simulink model "ServoTest"  (R2018a)
settings: Solver=VariableStepAuto  StartTime=0.0  StopTime=300  RelTol=1e-3
values from neighbouring files (symbols this model uses):
  s = mean(abs(present_speed.data))    [RunServoTest.m]
libraries: sm_lib x4, nesl_utility x4, powerlib_meascontrol x1
settings Model: Creator=matt  LastModifiedBy=matt
settings SolverCC: AlgebraicLoopSolver=LineSearch

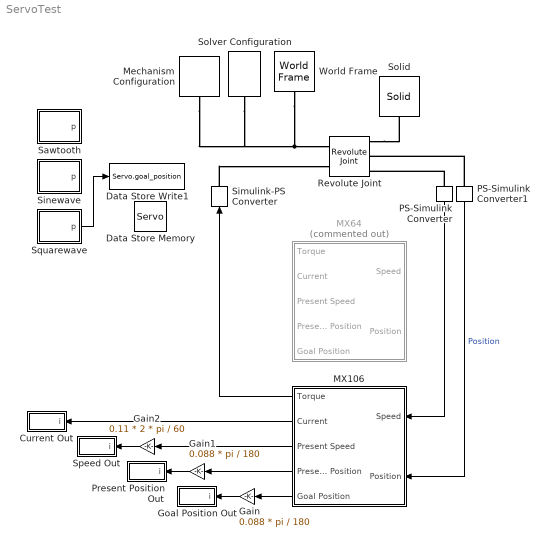
== system ServoTest ==
  Current Out : Subsystem
  Data Store Memory : DataStoreMemory  DataStoreName=Servo  ReadBeforeWriteMsg=warning  WriteAfterWriteMsg=warning  WriteAfterReadMsg=warning  InitialValue=MX64_default  ShowAdditionalParam=off  OutDataTypeStr=Bus: MX64_bus
  Data Store Write1 : DataStoreWrite  DataStoreName=Servo  DataStoreElements=Servo.goal_position
  Gain : Gain  Gain=0.088 * pi / 180
  Gain1 : Gain  Gain=0.088 * pi / 180
  Gain2 : Gain  Gain=0.11 * 2 * pi / 60
  Goal Position Out : Subsystem
  MX106 : Subsystem
  MX64 : Subsystem  Commented=on
  Mechanism Configuration : sm_lib/Utilities/Mechanism Configuration  UniformGravity=Constant  GravityVector=[0 0 0]  GravityUnits=m/s^2  LinearizationDelta=0.001
  PS-Simulink Converter : nesl_utility/PS-Simulink Converter  PhysicalDomain=network_engine_domain  SubClassName=ps_output  LeftPortType=input  RightPortType=output  PseudoPeriodic=off  Frequencies=[]  Unit=rad/s  AffineConversion=off
  PS-Simulink Converter1 : nesl_utility/PS-Simulink Converter  PhysicalDomain=network_engine_domain  SubClassName=ps_output  LeftPortType=input  RightPortType=output  PseudoPeriodic=off  Frequencies=[]  Unit=rad  AffineConversion=off
  Present Position Out : Subsystem
  Revolute Joint : sm_lib/Joints/Revolute Joint  SenseConstraintForce=off  SenseConstraintForceX=off  SenseConstraintForceY=off  SenseConstraintForceZ=off  SenseConstraintTorque=off  SenseConstraintTorqueX=off  SenseConstraintTorqueY=off  SenseConstraintTorqueZ=off  SenseTotalForce=off  SenseTotalForceX=off  SenseTotalForceY=off  SenseTotalForceZ=off  SenseTotalTorque=off  SenseTotalTorqueX=off  SenseTotalTorqueY=off  SenseTotalTorqueZ=off  CompositeWrenchDir=FollowerOnBase  CompositeWrenchFrame=BaseFrame  EquilibriumPosition=0  EquilibriumPositionUnits=deg  SpringStiffness=0  SpringStiffnessUnits=N*m/deg  DampingCoefficient=0  DampingCoefficientUnits=N*m/(rad/s)  TorqueActuationMode=InputTorque  MotionActuationMode=ComputedMotion  SensePosition=on  SenseVelocity=on  SenseAcceleration=off  SenseTorqueForce=off  PositionTargetSpecify=on  PositionTargetPriority=High  PositionTargetValue=MX64_init_position  PositionTargetValueUnits=deg  VelocityTargetSpecify=on  VelocityTargetPriority=High  VelocityTargetValue=MX64_init_speed  VelocityTargetValueUnits=deg/s
  Sawtooth : Subsystem
  Simulink-PS Converter : nesl_utility/Simulink-PS Converter  PhysicalDomain=network_engine_domain  SubClassName=ps_input  LeftPortType=input  RightPortType=output  PseudoPeriodic=off  Frequencies=[]  NoiseDistribution=none  NoiseParameters=[]  Unit=N*m  AffineConversion=off  FilteringAndDerivatives=provide  SimscapeFilterOrder=1  InputFilterTimeConstant=0.001  UdotUserProvided=0
  Sinewave : Subsystem
  Solid : sm_lib/Body Elements/Solid  InertiaType=CalculateFromGeometry  Mass=0.165  MassUnits=kg  CenterOfMass=[0 0 0]  CenterOfMassUnits=m  MomentsOfInertia=[1 1 1]  MomentsOfInertiaUnits=kg*m^2  ProductsOfInertia=[0 0 0]  ProductsOfInertiaUnits=kg*m^2  DensityBased=off  Density=1  DensityUnits=kg/m^3  DoExposeReferenceFrame=on  SerializedFrames=<Frames/>  GraphicType=FromGeometry  MarkerShape=Sphere  MarkerSize=10  GraphicVisPropType=SimpleVisualProperties  GraphicDiffuseColor=[0.5 0.5 0.5]  GraphicSpecularColor=[0.5 0.5 0.5 1.0]  GraphicAmbientColor=[0.15 0.15 0.15 1.0]  GraphicEmissiveColor=[0.0 0.0 0.0 1.0]  GraphicShininess=75  GraphicOpacity=1.0  GeometryShape=Brick  RectangleSize=[1 1]  RectangleSizeUnits=m  BrickDimensions=[1 1 1]  BrickDimensionUnits=m  CylinderRadius=1  CylinderRadiusUnits=m  CylinderLength=1  CylinderLengthUnits=m  SphereRadius=1  SphereRadiusUnits=m  EllipsoidRadii=[1 1 1]  EllipsoidRadiiUnits=m  ExtrusionCrossSection=[1 1; -1 1; -1 -1; 1 -1]  ExtrusionCrossSectionUnits=m  ExtrusionLength=1  ExtrusionLengthUnits=m  PolygonNumSides=3  PolygonOuterRadius=1  PolygonOuterRadiusUnits=m  ExtGeomFileType=STEP  ExtGeomFileUnits=m  RevolutionCrossSection=[1 1; 1 -1; 2 -1; 2 1]  RevolutionCrossSectionUnits=m  RevolutionExtent=Full  RevolutionAngle=180  RevolutionAngleUnits=deg
  Solver Configuration : nesl_utility/Solver Configuration  PhysicalDomain=network_engine_domain  SubClassName=solver  LeftPortType=input  RightPortType=generic  Tones=[]  Harmonics=[]  SimulateNoise=off  Profile=off  UseLocalSampling=off  EnableSwitchedLinearOptims=on  FrequencyDomain=off  UseCCode=off  RelTol=0.001  AbsTol=1e-06  MinStep=1e-09  ToWorkspace=off  RevertToSquareIcSolve=off  NumHomotopyIterations=100  PhasorMode=off  PhasorModeNumHarmonics=1  DoDC=off  ResidualTolerance=1e-09  UseLocalSolver=off  LocalSolverChoice=NE_BACKWARD_EULER_ADVANCER  LocalSolverSampleTime=0.001  DoFixedCost=off  MaxNonlinIter=3  MaxModeIter=2  LinearAlgebra=Sparse  EquationFormulation=NE_TIME_EF  DelaysMemoryBudget=1024  AutomaticFiltering=on  FilteringTimeConstant=0.001
  Speed Out : Subsystem
  Squarewave : Subsystem
  World Frame : sm_lib/Frames and Transforms/World Frame
  wires:
  Gain/1 -> Goal Position Out/1(i)
  Gain2/1 -> Speed Out/1(i)
  Gain1/1 -> Present Position Out/1(i)
  PS-Simulink Converter/1 -> MX106/1(Speed)
  PS-Simulink Converter1/1 -> MX106/2(Position)  "Position"
  MX106/1(Torque) -> Simulink-PS Converter/1
  MX106/2(Current) -> Current Out/1(i)
  MX106/3(Present Speed) -> Gain2/1
  MX106/4(Present Position) -> Gain1/1
  MX106/5(Goal Position) -> Gain/1
  Squarewave/1(p) -> Data Store Write1/1
  connections:
  World Frame/RConn1 -- Mechanism Configuration/RConn1 -- Solver Configuration/RConn1 -- Revolute Joint/LConn1
  Simulink-PS Converter/RConn1 -- Revolute Joint/LConn2
  PS-Simulink Converter/LConn1 -- Revolute Joint/RConn3
  Revolute Joint/RConn1 -- Solid/RConn1
  PS-Simulink Converter1/LConn1 -- Revolute Joint/RConn2

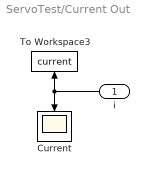
== system ServoTest/Current Out ==
  i : Inport
  Current : Scope
  To Workspace3 : ToWorkspace  VariableName=current  SaveFormat=Timeseries  SampleTime=-1
  wires:
  i/1 -> Current/1, To Workspace3/1

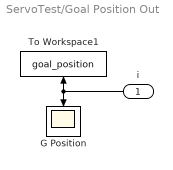
== system ServoTest/Goal Position Out ==
  i : Inport
  G Position : Scope
  To Workspace1 : ToWorkspace  VariableName=goal_position  SaveFormat=Timeseries  SampleTime=-1
  wires:
  i/1 -> G Position/1, To Workspace1/1

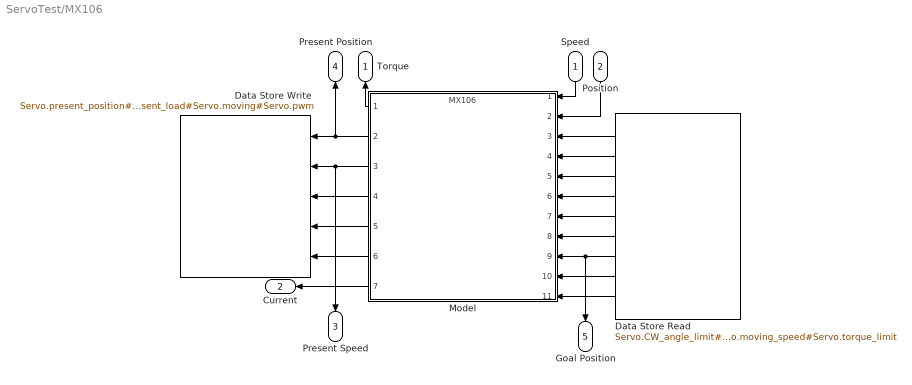
== system ServoTest/MX106 ==
  Speed : Inport
  Position : Inport  Port=2
  Data Store Read : DataStoreRead  DataStoreName=Servo  DataStoreElements=Servo.CW_angle_limit#Servo.CCW_angle_limit#Servo.torque_enable#Servo.D_gain#Servo.I_gain#Servo.P_gain#Servo.goal_position#Servo.moving_speed#Servo.torque_limit
  Data Store Write : DataStoreWrite  DataStoreName=Servo  DataStoreElements=Servo.present_position#Servo.present_speed#Servo.present_load#Servo.moving#Servo.pwm
  Model : ModelReference  ModelNameDialog=MX106  SimulationMode=Normal  ModelReferenceVersion=1.32
  Torque : Outport
  Current : Outport  Port=2
  Present Speed : Outport  Port=3
  Present Position : Outport  Port=4
  Goal Position : Outport  Port=5
  wires:
  Position/1 -> Model/2
  Data Store Read/5 -> Model/7
  Speed/1 -> Model/1
  Data Store Read/8 -> Model/10
  Data Store Read/3 -> Model/5
  Data Store Read/2 -> Model/4
  Model/3 -> Data Store Write/2, Present Speed/1
  Model/5 -> Data Store Write/4
  Model/6 -> Data Store Write/5
  Data Store Read/6 -> Model/8
  Model/2 -> Data Store Write/1, Present Position/1
  Data Store Read/9 -> Model/11
  Model/1 -> Torque/1
  Data Store Read/1 -> Model/3
  Model/7 -> Current/1
  Model/4 -> Data Store Write/3
  Data Store Read/7 -> Model/9, Goal Position/1
  Data Store Read/4 -> Model/6

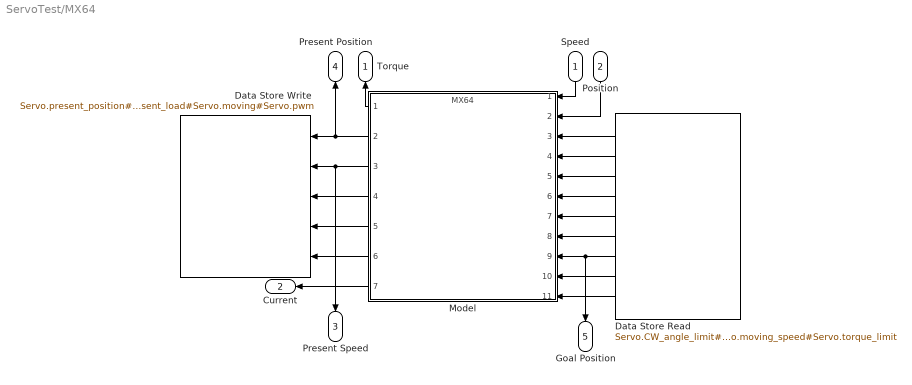
== system ServoTest/MX64 ==
  Speed : Inport
  Position : Inport  Port=2
  Data Store Read : DataStoreRead  DataStoreName=Servo  DataStoreElements=Servo.CW_angle_limit#Servo.CCW_angle_limit#Servo.torque_enable#Servo.D_gain#Servo.I_gain#Servo.P_gain#Servo.goal_position#Servo.moving_speed#Servo.torque_limit
  Data Store Write : DataStoreWrite  DataStoreName=Servo  DataStoreElements=Servo.present_position#Servo.present_speed#Servo.present_load#Servo.moving#Servo.pwm
  Model : ModelReference  ModelNameDialog=MX64  SimulationMode=Normal  ModelReferenceVersion=1.27
  Torque : Outport
  Current : Outport  Port=2
  Present Speed : Outport  Port=3
  Present Position : Outport  Port=4
  Goal Position : Outport  Port=5
  wires:
  Position/1 -> Model/2
  Data Store Read/5 -> Model/7
  Speed/1 -> Model/1
  Data Store Read/8 -> Model/10
  Data Store Read/3 -> Model/5
  Data Store Read/2 -> Model/4
  Model/3 -> Data Store Write/2, Present Speed/1
  Model/5 -> Data Store Write/4
  Model/6 -> Data Store Write/5
  Data Store Read/6 -> Model/8
  Model/2 -> Data Store Write/1, Present Position/1
  Data Store Read/9 -> Model/11
  Model/1 -> Torque/1
  Data Store Read/1 -> Model/3
  Model/7 -> Current/1
  Model/4 -> Data Store Write/3
  Data Store Read/7 -> Goal Position/1, Model/9
  Data Store Read/4 -> Model/6

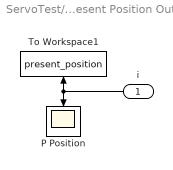
== system ServoTest/Present Position Out ==
  i : Inport
  P Position : Scope
  To Workspace1 : ToWorkspace  VariableName=present_position  SaveFormat=Timeseries  SampleTime=-1
  wires:
  i/1 -> P Position/1, To Workspace1/1

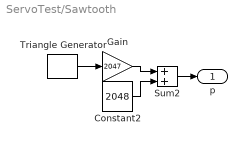
== system ServoTest/Sawtooth ==
  Constant2 : Constant  Value=2048
  Gain : Gain  Gain=2047
  Sum2 : Sum  OutDataTypeStr=int16
  Triangle Generator : powerlib_meascontrol/Pulse & Signal Generators/Triangle Generator  Freq=1 / 206  Phase=0  Ts=0
  p : Outport
  wires:
  Constant2/1 -> Sum2/2
  Triangle Generator/1 -> Gain/1
  Sum2/1 -> p/1
  Gain/1 -> Sum2/1

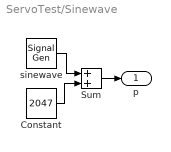
== system ServoTest/Sinewave ==
  Constant : Constant  Value=2047
  Sum : Sum  OutDataTypeStr=int16
  sinewave : SignalGenerator  Amplitude=2047  Frequency=2 * pi / 150  Units=rad/sec
  p : Outport
  wires:
  sinewave/1 -> Sum/1
  Constant/1 -> Sum/2
  Sum/1 -> p/1

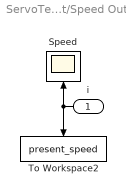
== system ServoTest/Speed Out ==
  i : Inport
  Speed : Scope
  To Workspace2 : ToWorkspace  VariableName=present_speed  SaveFormat=Timeseries  SampleTime=-1
  wires:
  i/1 -> To Workspace2/1, Speed/1

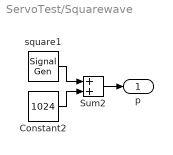
== system ServoTest/Squarewave ==
  Constant2 : Constant  Value=1024
  Sum2 : Sum  OutDataTypeStr=int16
  square1 : SignalGenerator  WaveForm=square  Amplitude=1024  Frequency=2 * pi / 100  Units=rad/sec
  p : Outport
  wires:
  Constant2/1 -> Sum2/2
  square1/1 -> Sum2/1
  Sum2/1 -> p/1
